simulink model "test_condenser"  (R2021b)
settings: Solver=VariableStepAuto  StartTime=0.0  StopTime=10.0  RelTol=1e-3
settings Model: Creator=Edwar  LastModifiedBy=Edwar

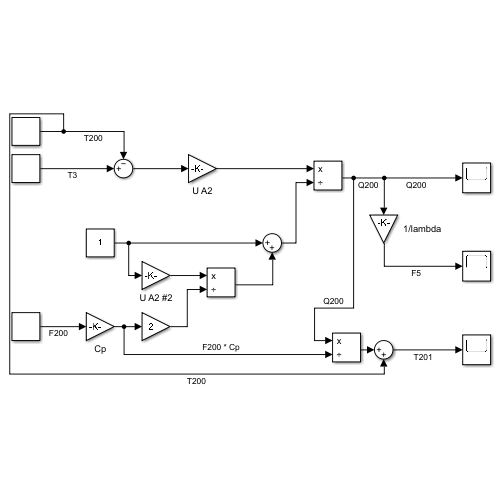
[thumbnail: Simulink's stored preview of the top-level diagram]
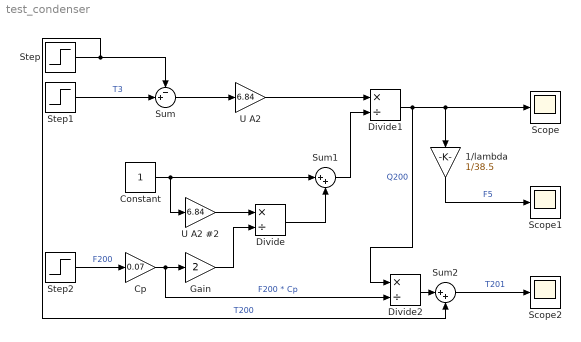
== system test_condenser ==
  1/lambda : Gain  Gain=1/38.5
  Constant : Constant
  Cp : Gain  Gain=0.07
  Divide : Product  Inputs=*/
  Divide1 : Product  Inputs=*/
  Divide2 : Product  Inputs=*/
  Gain : Gain  Gain=2
  Scope : Scope
  Scope1 : Scope
  Scope2 : Scope
  Step : Step  SampleTime=0
  Step1 : Step  Before=1  After=2  SampleTime=0
  Step2 : Step  SampleTime=0
  Sum : Sum  Inputs=-+|
  Sum1 : Sum  Inputs=|++
  Sum2 : Sum  Inputs=|++
  U A2 : Gain  Gain=6.84
  U A2 #2 : Gain  Gain=6.84
  wires:
  Sum/1 -> U A2/1
  Constant/1 -> U A2 #2/1, Sum1/1
  Gain/1 -> Divide/2
  U A2 #2/1 -> Divide/1
  Divide/1 -> Sum1/2
  U A2/1 -> Divide1/1
  Sum1/1 -> Divide1/2
  Divide1/1 -> Divide2/1, Scope/1, 1/lambda/1  "Q200"
  Step1/1 -> Sum/2  "T3"
  Step/1 -> Sum2/2, Sum/1  "T200"
  Cp/1 -> Divide2/2, Gain/1  "F200 * Cp"
  Step2/1 -> Cp/1  "F200"
  Divide2/1 -> Sum2/1
  Sum2/1 -> Scope2/1  "T201"
  1/lambda/1 -> Scope1/1  "F5"
